simulink model "mech_transmission"  (Simulink 6.0)
settings: Solver=ode45  StartTime=0.0  StopTime=100  RelTol=1e-4  AbsTol=1e-4
PreLoadFcn:
  | load mech_transmission_data;
undefined symbols (not defined in the file or in its folder): converter_data, downtab, emap, Iei, Iint, mutable, Nf, r1, r2, radvec, thvec, uptab, vehicledata
libraries: mblibv1 x64
(part 2 of 2)

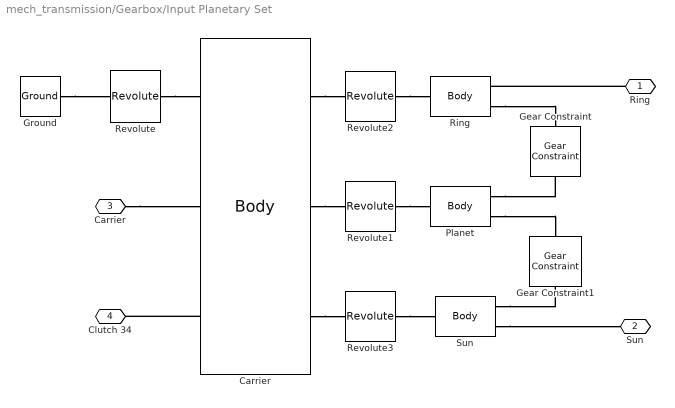
== system mech_transmission/Gearbox/Input Planetary Set ==
  Carrier : mblibv1/Bodies/Body  Tag=Factory generic  Description=Mechanical Blockset  PhysicalDomain=mechanical  SubClassName=Unknown  LeftPortType=workingframe  RightPortType=workingframe  LConnTagsString=CS1|CS5|CS6  RConnTagsString=CS2|CS3|CS4  DialogClass=MechanicalBodyBlock  Mass=0  MassUnits=kg  InertiaUnits=kg*m^2  Inertia=diag([0 0 Ic])  Shape=Cylinder  ShapeDims=[1 1]  ShapeUnits=m  ShapeUse=false  Density=1  DensityUnits=kg/m^3  DensityUse=false  CG=Left$CG$[0 0 0]$WORLD$WORLD$m$[0 0 0]$Euler X-Y-Z$deg$WORLD$false  WorkingFrames=Left$CS1$[0 0 0]$CG$CG$m$[0 0 0]$Euler X-Y-Z$deg$WORLD$true#Left$CS5$[0 0 0]$CG$CG$m$[0 0 0]$Euler X-Y-Z$deg$WORLD$true#Left$CS6$[0 0 0]$CG$CG$m$[0 0 0]$Euler X-Y-Z$deg$WORLD$true#Right$CS2$[0 0 0]$CG$CG$m$[0 0 0]$Euler X-Y-Z$deg$WORLD$true#Right$CS3$[(1+R)/2 0 0]$CG$CG$m$[0 0 0]$Euler X-Y-Z$deg$WORLD$true#Right$CS4$[0 0 0]$CG$CG$m$[0 0 0]$Euler X-Y-Z$deg$WORLD$true
  Gear Constraint : mblibv1/Constraints &  Drivers/Gear Constraint  Tag=Factory generic  Description=Mechanical Blockset  Orientation=down  PhysicalDomain=mechanical  SubClassName=Unknown  LeftPortType=blob  RightPortType=blob  LConnTagsString=__newl0  RConnTagsString=__newr0  DialogClass=GearConstraint  NumSAPorts=0  BaseRadius=R  BaseRadiusUnits=m  FollowerRadius=(R-1)/2  FollowerRadiusUnits=m
  Gear Constraint1 : mblibv1/Constraints &  Drivers/Gear Constraint  Tag=Factory generic  Description=Mechanical Blockset  Orientation=up  PhysicalDomain=mechanical  SubClassName=Unknown  LeftPortType=blob  RightPortType=blob  LConnTagsString=__newl0  RConnTagsString=__newr0  DialogClass=GearConstraint  NumSAPorts=0  BaseRadius=1  BaseRadiusUnits=m  FollowerRadius=(R-1)/2  FollowerRadiusUnits=m
  Ground : mblibv1/Bodies/Ground  Opaque=on  LeftPortType=env  RightPortType=workingframe  PhysicalDomain=Mechanical  DialogClass=GroundBlock  CoordPosition=[0 0 0]  CoordPositionUnits=m  StateVectorMgrId=-1  MachineId=[0 0]  ShowEnvPort=off
  Planet : mblibv1/Bodies/Body  Tag=Factory generic  Description=Mechanical Blockset  PhysicalDomain=mechanical  SubClassName=Unknown  LeftPortType=workingframe  RightPortType=workingframe  LConnTagsString=CS1  RConnTagsString=CS2|CS3  DialogClass=MechanicalBodyBlock  Mass=0  MassUnits=kg  InertiaUnits=kg*m^2  Inertia=diag([0 0 Ip])  Shape=Cylinder  ShapeDims=[1 1]  ShapeUnits=m  ShapeUse=false  Density=1  DensityUnits=kg/m^3  DensityUse=false  CG=Left$CG$[0 0 0]$WORLD$WORLD$m$[0 0 0]$Euler X-Y-Z$deg$WORLD$false  WorkingFrames=Left$CS1$[(1+R)/2 0 0]$WORLD$WORLD$m$[0 0 0]$Euler X-Y-Z$deg$WORLD$true#Right$CS2$[0 0 0]$CS1$CS1$m$[0 0 0]$Euler X-Y-Z$deg$WORLD$true#Right$CS3$[0 0 0]$CS1$CS1$m$[0 0 0]$Euler X-Y-Z$deg$WORLD$true
  Revolute : mblibv1/Joints/Revolute  Tag=Factory generic  Description=Mechanical Blockset  PhysicalDomain=mechanical  SubClassName=Unknown  LeftPortType=blob  RightPortType=blob  LConnTagsString=__newl0  RConnTagsString=__newr0  NumSAPorts=0  CutJoint=off  MarkAsCut=off  Primitives=revolute  PrimitiveProps=R1$WORLD$[0 0 1]$revolute  DialogClass=JointBlock
  Revolute1 : mblibv1/Joints/Revolute  Tag=Factory generic  Description=Mechanical Blockset  PhysicalDomain=mechanical  SubClassName=Unknown  LeftPortType=blob  RightPortType=blob  LConnTagsString=__newl0  RConnTagsString=__newr0  NumSAPorts=0  CutJoint=off  MarkAsCut=off  Primitives=revolute  PrimitiveProps=R1$INERTIAL$[0 0 1]$revolute  DialogClass=JointBlock
  Revolute2 : mblibv1/Joints/Revolute  Tag=Factory generic  Description=Mechanical Blockset  PhysicalDomain=mechanical  SubClassName=Unknown  LeftPortType=blob  RightPortType=blob  LConnTagsString=__newl0  RConnTagsString=__newr0  NumSAPorts=0  CutJoint=off  MarkAsCut=off  Primitives=revolute  PrimitiveProps=R1$INERTIAL$[0 0 1]$revolute  DialogClass=JointBlock
  Revolute3 : mblibv1/Joints/Revolute  Tag=Factory generic  Description=Mechanical Blockset  PhysicalDomain=mechanical  SubClassName=Unknown  LeftPortType=blob  RightPortType=blob  LConnTagsString=__newl0  RConnTagsString=__newr0  NumSAPorts=0  CutJoint=off  MarkAsCut=off  Primitives=revolute  PrimitiveProps=R1$INERTIAL$[0 0 1]$revolute  DialogClass=JointBlock
  Ring : mblibv1/Bodies/Body  Tag=Factory generic  Description=Mechanical Blockset  PhysicalDomain=mechanical  SubClassName=Unknown  LeftPortType=workingframe  RightPortType=workingframe  LConnTagsString=CS1  RConnTagsString=CS2|CS3  DialogClass=MechanicalBodyBlock  Mass=0  MassUnits=kg  InertiaUnits=kg*m^2  Inertia=diag([0 0 Ir])  Shape=Cylinder  ShapeDims=[1 1]  ShapeUnits=m  ShapeUse=false  Density=1  DensityUnits=kg/m^3  DensityUse=false  CG=Left$CG$[0 0 0]$WORLD$WORLD$m$[0 0 0]$Euler X-Y-Z$deg$WORLD$false  WorkingFrames=Left$CS1$[0 0 0]$CG$CG$m$[0 0 0]$Euler X-Y-Z$deg$WORLD$true#Right$CS2$[0 0 0]$CG$CG$m$[0 0 0]$Euler X-Y-Z$deg$WORLD$true#Right$CS3$[0 0 0]$CG$CG$m$[0 0 0]$Euler X-Y-Z$deg$WORLD$true
  Sun : mblibv1/Bodies/Body  Tag=Factory generic  Description=Mechanical Blockset  PhysicalDomain=mechanical  SubClassName=Unknown  LeftPortType=workingframe  RightPortType=workingframe  LConnTagsString=CS1  RConnTagsString=CS2|CS3  DialogClass=MechanicalBodyBlock  Mass=0  MassUnits=kg  InertiaUnits=kg*m^2  Inertia=diag([0 0 Is])  Shape=Cylinder  ShapeDims=[1 1]  ShapeUnits=m  ShapeUse=false  Density=1  DensityUnits=kg/m^3  DensityUse=false  CG=Left$CG$[0 0 0]$WORLD$WORLD$m$[0 0 0]$Euler X-Y-Z$deg$WORLD$false  WorkingFrames=Left$CS1$[0 0 0]$WORLD$WORLD$m$[0 0 0]$Euler X-Y-Z$deg$WORLD$true#Right$CS2$[0 0 0]$WORLD$WORLD$m$[0 0 0]$Euler X-Y-Z$deg$WORLD$true#Right$CS3$[0 0 0]$WORLD$WORLD$m$[0 0 0]$Euler X-Y-Z$deg$WORLD$true
  "Ring " : PMIOPort  Orientation=left  Port=1  Side=Right
  "Sun  " : PMIOPort  Orientation=left  Port=2  Side=Right
  "Carrier " : PMIOPort  Port=3  Side=Left
  Clutch 34 : PMIOPort  Port=4  Side=Right
  connections:
  Ground/RConn1 -- Revolute/LConn1
  Revolute/RConn1 -- Carrier/LConn1
  Revolute1/RConn1 -- Planet/LConn1
  Carrier/RConn2 -- Revolute1/LConn1
  Carrier/RConn1 -- Revolute2/LConn1
  Carrier/RConn3 -- Revolute3/LConn1
  Revolute2/RConn1 -- Ring/LConn1
  Revolute3/RConn1 -- Sun/LConn1
  "Ring "/RConn1 -- Ring/RConn1
  "Carrier "/RConn1 -- Carrier/LConn2
  Sun/RConn2 -- "Sun  "/RConn1
  Carrier/LConn3 -- Clutch 34/RConn1
  Ring/RConn2 -- Gear Constraint/LConn1
  Planet/RConn1 -- Gear Constraint/RConn1
  Planet/RConn2 -- Gear Constraint1/RConn1
  Sun/RConn1 -- Gear Constraint1/LConn1

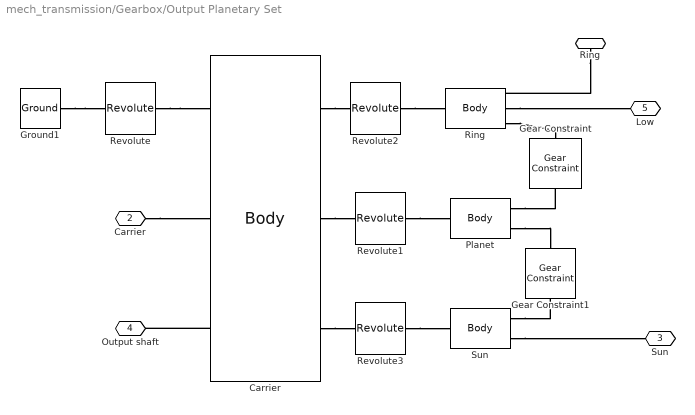
== system mech_transmission/Gearbox/Output Planetary Set ==
  Carrier : mblibv1/Bodies/Body  Tag=Factory generic  Description=Mechanical Blockset  PhysicalDomain=mechanical  SubClassName=Unknown  LeftPortType=workingframe  RightPortType=workingframe  LConnTagsString=CS1|CS5|CS6  RConnTagsString=CS2|CS3|CS4  DialogClass=MechanicalBodyBlock  Mass=0  MassUnits=kg  InertiaUnits=kg*m^2  Inertia=[0 0 0;0 0 0;0 0 Ic]  Shape=Cylinder  ShapeDims=[1 1]  ShapeUnits=m  ShapeUse=false  Density=1  DensityUnits=kg/m^3  DensityUse=false  CG=Left$CG$[0 0 0]$WORLD$WORLD$m$[0 0 0]$Euler X-Y-Z$deg$WORLD$false  WorkingFrames=Left$CS1$[0 0 0]$CG$CG$m$[0 0 0]$Euler X-Y-Z$deg$WORLD$true#Left$CS5$[0 0 0]$CG$CG$m$[0 0 0]$Euler X-Y-Z$deg$WORLD$true#Left$CS6$[0 0 0]$CG$CG$m$[0 0 0]$Euler X-Y-Z$deg$WORLD$true#Right$CS2$[0 0 0]$CG$CG$m$[0 0 0]$Euler X-Y-Z$deg$WORLD$true#Right$CS3$[(1+R)/2 0 0]$CG$CG$m$[0 0 0]$Euler X-Y-Z$deg$WORLD$true#Right$CS4$[0 0 0]$CG$CG$m$[0 0 0]$Euler X-Y-Z$deg$WORLD$true
  Gear Constraint : mblibv1/Constraints &  Drivers/Gear Constraint  Tag=Factory generic  Description=Mechanical Blockset  Orientation=down  PhysicalDomain=mechanical  SubClassName=Unknown  LeftPortType=blob  RightPortType=blob  LConnTagsString=__newl0  RConnTagsString=__newr0  DialogClass=GearConstraint  NumSAPorts=0  BaseRadius=R  BaseRadiusUnits=m  FollowerRadius=(R-1)/2  FollowerRadiusUnits=m
  Gear Constraint1 : mblibv1/Constraints &  Drivers/Gear Constraint  Tag=Factory generic  Description=Mechanical Blockset  Orientation=up  PhysicalDomain=mechanical  SubClassName=Unknown  LeftPortType=blob  RightPortType=blob  LConnTagsString=__newl0  RConnTagsString=__newr0  DialogClass=GearConstraint  NumSAPorts=0  BaseRadius=1  BaseRadiusUnits=m  FollowerRadius=(R-1)/2  FollowerRadiusUnits=m
  Ground1 : mblibv1/Bodies/Ground  Opaque=on  LeftPortType=env  RightPortType=workingframe  PhysicalDomain=Mechanical  DialogClass=GroundBlock  CoordPosition=[0 0 0]  CoordPositionUnits=m  StateVectorMgrId=-1  MachineId=[0 0]  ShowEnvPort=off
  Planet : mblibv1/Bodies/Body  Tag=Factory generic  Description=Mechanical Blockset  PhysicalDomain=mechanical  SubClassName=Unknown  LeftPortType=workingframe  RightPortType=workingframe  LConnTagsString=CS1  RConnTagsString=CS2|CS3  DialogClass=MechanicalBodyBlock  Mass=0  MassUnits=kg  InertiaUnits=kg*m^2  Inertia=[0 0 0;0 0 0;0 0 Ip]  Shape=Cylinder  ShapeDims=[1 1]  ShapeUnits=m  ShapeUse=false  Density=1  DensityUnits=kg/m^3  DensityUse=false  CG=Left$CG$[0 0 0]$WORLD$WORLD$m$[0 0 0]$Euler X-Y-Z$deg$WORLD$false  WorkingFrames=Left$CS1$[(1+R)/2 0 0]$WORLD$WORLD$m$[0 0 0]$Euler X-Y-Z$deg$WORLD$true#Right$CS2$[0 0 0]$CS1$CS1$m$[0 0 0]$Euler X-Y-Z$deg$WORLD$true#Right$CS3$[0 0 0]$CS1$CS1$m$[0 0 0]$Euler X-Y-Z$deg$WORLD$true
  Revolute{,1..3} (4 alike) : mblibv1/Joints/Revolute  Tag=Factory generic  Description=Mechanical Blockset  PhysicalDomain=mechanical  SubClassName=Unknown  LeftPortType=blob  RightPortType=blob  LConnTagsString=__newl0  RConnTagsString=__newr0  NumSAPorts=0  CutJoint=off  MarkAsCut=off  Primitives=revolute  PrimitiveProps=R1$WORLD$[0 0 1]$revolute  DialogClass=JointBlock
  Ring : mblibv1/Bodies/Body  Tag=Factory generic  Description=Mechanical Blockset  PhysicalDomain=mechanical  SubClassName=Unknown  LeftPortType=workingframe  RightPortType=workingframe  LConnTagsString=CS1  RConnTagsString=CS2|CS4|CS3  DialogClass=MechanicalBodyBlock  Mass=0  MassUnits=kg  InertiaUnits=kg*m^2  Inertia=[0 0 0;0 0 0;0 0 Ir]  Shape=Cylinder  ShapeDims=[1 1]  ShapeUnits=m  ShapeUse=false  Density=1  DensityUnits=kg/m^3  DensityUse=false  CG=Left$CG$[0 0 0]$WORLD$WORLD$m$[0 0 0]$Euler X-Y-Z$deg$WORLD$false  WorkingFrames=Left$CS1$[0 0 0]$CG$CG$m$[0 0 0]$Euler X-Y-Z$deg$WORLD$true#Right$CS2$[0 0 0]$CG$CG$m$[0 0 0]$Euler X-Y-Z$deg$WORLD$true#Right$CS4$[0 0 0]$CG$CG$m$[0 0 0]$Euler X-Y-Z$deg$WORLD$true#Right$CS3$[0 0 0]$CG$CG$m$[0 0 0]$Euler X-Y-Z$deg$WORLD$true
  Sun : mblibv1/Bodies/Body  Tag=Factory generic  Description=Mechanical Blockset  PhysicalDomain=mechanical  SubClassName=Unknown  LeftPortType=workingframe  RightPortType=workingframe  LConnTagsString=CS1  RConnTagsString=CS2|CS3  DialogClass=MechanicalBodyBlock  Mass=0  MassUnits=kg  InertiaUnits=kg*m^2  Inertia=[0 0 0;0 0 0;0 0 Is]  Shape=Cylinder  ShapeDims=[1 1]  ShapeUnits=m  ShapeUse=false  Density=1  DensityUnits=kg/m^3  DensityUse=false  CG=Left$CG$[0 0 0]$WORLD$WORLD$m$[0 0 0]$Euler X-Y-Z$deg$WORLD$false  WorkingFrames=Left$CS1$[0 0 0]$WORLD$WORLD$m$[0 0 0]$Euler X-Y-Z$deg$WORLD$true#Right$CS2$[0 0 0]$WORLD$WORLD$m$[0 0 0]$Euler X-Y-Z$deg$WORLD$true#Right$CS3$[0 0 0]$WORLD$WORLD$m$[0 0 0]$Euler X-Y-Z$deg$WORLD$true
  "Ring " : PMIOPort  Orientation=down  Port=1  Side=Right
  "Carrier " : PMIOPort  Port=2  Side=Left
  "Sun " : PMIOPort  Orientation=left  Port=3  Side=Right
  Output shaft : PMIOPort  Port=4  Side=Left
  Low : PMIOPort  Orientation=left  Port=5  Side=Right
  connections:
  Sun/RConn2 -- "Sun "/RConn1
  "Carrier "/RConn1 -- Carrier/LConn2
  "Ring "/RConn1 -- Ring/RConn1
  Revolute3/RConn1 -- Sun/LConn1
  Revolute2/RConn1 -- Ring/LConn1
  Carrier/RConn3 -- Revolute3/LConn1
  Carrier/RConn1 -- Revolute2/LConn1
  Carrier/RConn2 -- Revolute1/LConn1
  Revolute1/RConn1 -- Planet/LConn1
  Revolute/RConn1 -- Carrier/LConn1
  Ground1/RConn1 -- Revolute/LConn1
  Ring/RConn2 -- Low/RConn1
  Carrier/LConn3 -- Output shaft/RConn1
  Ring/RConn3 -- Gear Constraint/LConn1
  Planet/RConn1 -- Gear Constraint/RConn1
  Planet/RConn2 -- Gear Constraint1/RConn1
  Sun/RConn1 -- Gear Constraint1/LConn1

== system mech_transmission/Turbine/Torbine torque ==
  Torque : Inport  Port=1  LatchInput=off
  Body Actuator : mblibv1/Sensors &  Actuators/Body Actuator  Description=Mechanical Blockset  Orientation=up  Opaque=on  PhysicalDomain=Mechanical  PortType=blob  ActuationStyle=Force  AngleUnits=deg  ArcVelocityUnits=deg/s  ArcAccelerationUnits=deg/s^2  CoordPositionUnits=m  VelocityUnits=m/s  AccelerationUnits=m/s^2  ForceUnits=N  TorqueUnits=N-m  ActiveIO=on  Width=3  DialogClass=MechanicalActuatorBlock  ReferenceFrame=Absolute (World)  Angle=off  CoordPosition=on  Force=off  Torque=on
  Constant : Constant  Value=0
  Mux : Mux  Inputs=3
  Turbine : PMIOPort  Orientation=down  Port=1  Side=Right
  wires:
  Mux/1 -> Body Actuator/1
  Torque/1 -> Mux/3
  Constant/1 -> Mux/1, Mux/2
  connections:
  Turbine/RConn1 -- Body Actuator/RConn1

== stateflow chart  Shift_logic ==
  settings: updateMethod=DISCRETE  sampleTime=0.04
  state gear_selection/
    state gear_state [parallel]
      state fourth/
        entry: gear = 4;
      state third/
        entry: gear = 3;
      state second/
        entry: gear = 2;
      state first/
        entry: gear = 1;
      third -> fourth : UPSHIFT34
      first -> second : UPSHIFT12
      second -> third : UPSHIFT23
      (default) -> first
      fourth -> third : DOWNSHIFT43
      third -> second : DOWNSHIFT32
      second -> first : DOWNSHIFT21
    state selection_state/ [parallel]
      during: compute_thresholds;
      state downshift_confirm/
        entry: tdn = t;
      state upshift_confirm/
        entry: tup = t;
      state steady_state
      (default) -> steady_state
      steady_state -> downshift_confirm : [vehicle_speed < down_threshold]
      steady_state -> upshift_confirm : [vehicle_speed > up_threshold]
      downshift_confirm -> steady_state : [vehicle_speed > down_threshold]
      (junction 13) -> steady_state
      (junction 14) -> steady_state
      upshift_confirm -> steady_state : [vehicle_speed < up_threshold]
      upshift_confirm -> (junction 16) : [t - tup >= Tconfirm & ...
          | vehicle_speed >= up_threshold]
      downshift_confirm -> (junction 15) : [t - tdn >= Tconfirm & ...
          | vehicle_speed <= down_threshold]
      (junction 15) -> (junction 13) : [gear ==4]/DOWNSHIFT43
      (junction 16) -> (junction 14) : [gear == 3]{UPSHIFT34}
      (junction 15) -> (junction 13) : [gear == 3]/DOWNSHIFT32
      (junction 16) -> (junction 14) : [gear == 2]{UPSHIFT23}
      (junction 15) -> (junction 13) : [gear == 2]/DOWNSHIFT21
      (junction 16) -> (junction 14) : [gear == 1]{UPSHIFT12}
  data: gear output double size=1 [1..4] =1; tdn local double size=1; tup local double size=1; Tconfirm parameter double size=1; down_threshold input double size=1; up_threshold input double size=1; vehicle_speed input double size=1
  data gear settings: units=int
  data vehicle_speed settings: units=double
  events: UPSHIFT12 local EITHER_EDGE_EVENT; UPSHIFT23 local EITHER_EDGE_EVENT; UPSHIFT34 local EITHER_EDGE_EVENT; DOWNSHIFT21 local EITHER_EDGE_EVENT; DOWNSHIFT32 local EITHER_EDGE_EVENT; DOWNSHIFT43 local EITHER_EDGE_EVENT; compute_thresholds output FUNCTION_CALL_EVENT
